simulink model "clutch"  (R2020a)
settings: Solver=VariableStepAuto  StartTime=0.0  StopTime=10.0  RelTol=1e-3
PostLoadFcn:
  | Fn=[0 0;1 0.8;2 1.6;3 1.6;4 1.6;5 1.6;6 0.8;7 0;8 0;9 0;10 0];
  | muk=1;
  | mus=1.5;
  | R=1;
  | Tin=[1 2;2 2;3 2;4 2;5 2;6 0;7 0;8 0;9 0;10 0];
  | Ie=1;
  | be=2;
  | Iv=5;
  | bv=1;
settings Model: Creator=Hp  LastModifiedBy=Hp

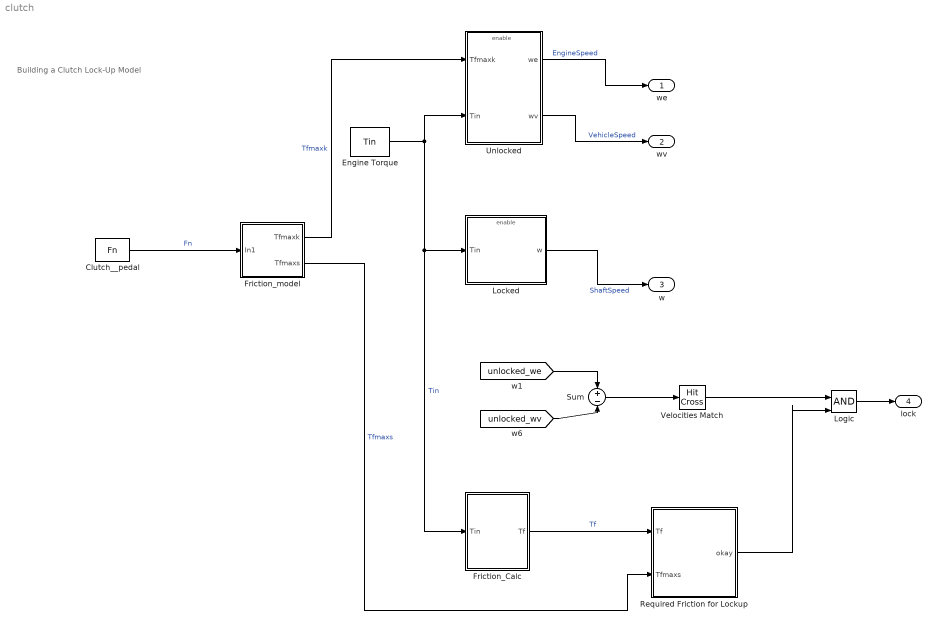
== system clutch ==
  note: Building a Clutch Lock-Up Model
  Clutch__pedal : FromWorkspace  VariableName=Fn
  Engine Torque : FromWorkspace  VariableName=Tin
  Friction_Calc : Subsystem
  Friction_model : Subsystem
  Locked : Subsystem
  Logic : Logic  IconShape=distinctive  OutDataTypeStr=boolean
  Required Friction for Lockup : Subsystem
  Sum : Sum  Inputs=+-  InputSameDT=on  SaturateOnIntegerOverflow=on  OutDataTypeStr=Inherit: Same as first input
  Unlocked : Subsystem
  Velocities Match : HitCross
  we : Outport  InitialOutput=0  VectorParamsAs1DForOutWhenUnconnected=off
  wv : Outport  Port=2  InitialOutput=0  VectorParamsAs1DForOutWhenUnconnected=off
  w : Outport  Port=3  InitialOutput=0  VectorParamsAs1DForOutWhenUnconnected=off
  lock : Outport  Port=4  InitialOutput=0  VectorParamsAs1DForOutWhenUnconnected=off
  wires:
  Clutch__pedal/1 -> Friction_model/1(In1)  "Fn"
  Engine Torque/1 -> Locked/1(Tin), Friction_Calc/1(Tin), Unlocked/2(Tin)  "Tin"
  Friction_model/1(Tfmaxk) -> Unlocked/1(Tfmaxk)  "Tfmaxk"
  Unlocked/1(we) -> we/1  "EngineSpeed"
  Unlocked/2(wv) -> wv/1  "VehicleSpeed"
  Locked/1(w) -> w/1  "ShaftSpeed"
  [unlocked_we] -> Sum/1
  Sum/1 -> Velocities Match/1
  Logic/1 -> lock/1
  [unlocked_wv] -> Sum/2
  Velocities Match/1 -> Logic/1
  Friction_model/2(Tfmaxs) -> Required Friction for Lockup/2(Tfmaxs)  "Tfmaxs"
  Friction_Calc/1(Tf) -> Required Friction for Lockup/1(Tf)  "Tf"
  Required Friction for Lockup/1(okay) -> Logic/2

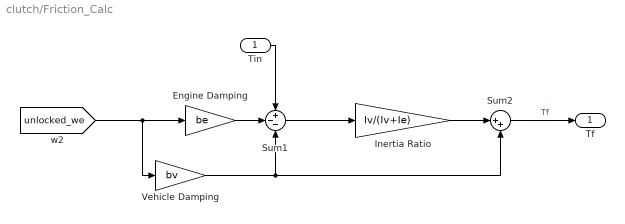
== system clutch/Friction_Calc ==
  Tin : Inport
  Engine Damping : Gain  Gain=be  SaturateOnIntegerOverflow=on  OutDataTypeStr=Inherit: Same as input  ParamDataTypeStr=Inherit: Same as input
  Inertia Ratio : Gain  Gain=Iv/(Iv+Ie)  SaturateOnIntegerOverflow=on  OutDataTypeStr=Inherit: Same as input  ParamDataTypeStr=Inherit: Same as input
  Sum1 : Sum  Inputs=+--  InputSameDT=on  SaturateOnIntegerOverflow=on  OutDataTypeStr=Inherit: Same as first input
  Sum2 : Sum  Inputs=|++  InputSameDT=on  SaturateOnIntegerOverflow=on  OutDataTypeStr=Inherit: Same as first input
  Vehicle Damping : Gain  Gain=bv  SaturateOnIntegerOverflow=on  OutDataTypeStr=Inherit: Same as input  ParamDataTypeStr=Inherit: Same as input
  Tf : Outport
  wires:
  Tin/1 -> Sum1/1
  [unlocked_we] -> Vehicle Damping/1, Engine Damping/1
  Inertia Ratio/1 -> Sum2/1
  Sum1/1 -> Inertia Ratio/1
  Sum2/1 -> Tf/1  "Tf"
  Engine Damping/1 -> Sum1/2
  Vehicle Damping/1 -> Sum2/2, Sum1/3

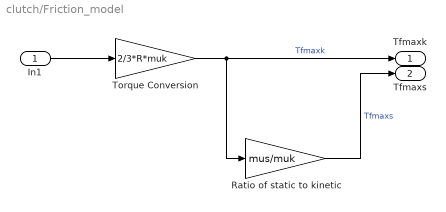
== system clutch/Friction_model ==
  In1 : Inport
  Ratio of static to kinetic : Gain  Gain=mus/muk  SaturateOnIntegerOverflow=on  OutDataTypeStr=Inherit: Same as input  ParamDataTypeStr=Inherit: Same as input
  Torque Conversion : Gain  Gain=2/3*R*muk  SaturateOnIntegerOverflow=on  OutDataTypeStr=Inherit: Same as input  ParamDataTypeStr=Inherit: Same as input
  Tfmaxk : Outport
  Tfmaxs : Outport  Port=2
  wires:
  In1/1 -> Torque Conversion/1
  Torque Conversion/1 -> Tfmaxk/1, Ratio of static to kinetic/1  "Tfmaxk"
  Ratio of static to kinetic/1 -> Tfmaxs/1  "Tfmaxs"

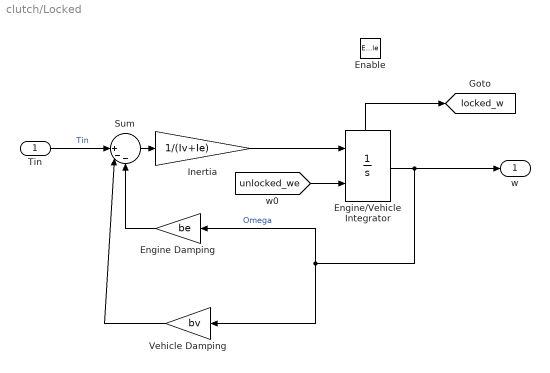
== system clutch/Locked ==
  Tin : Inport
  Enable : EnablePort
  Engine Damping : Gain  Gain=be  SaturateOnIntegerOverflow=on  OutDataTypeStr=Inherit: Same as input  ParamDataTypeStr=Inherit: Same as input
  Engine/Vehicle Integrator : Integrator  InitialConditionSource=external  ShowStatePort=on
  Inertia : Gain  Gain=1/(Iv+Ie)  SaturateOnIntegerOverflow=on  OutDataTypeStr=Inherit: Same as input  ParamDataTypeStr=Inherit: Same as input
  Sum : Sum  Inputs=||+--  InputSameDT=on  SaturateOnIntegerOverflow=on  OutDataTypeStr=Inherit: Same as first input
  Vehicle Damping : Gain  Gain=bv  SaturateOnIntegerOverflow=on  OutDataTypeStr=Inherit: Same as input  ParamDataTypeStr=Inherit: Same as input
  w : Outport  InitialOutput=0  VectorParamsAs1DForOutWhenUnconnected=off
  tag scope: locked_w=global
  wires:
  Inertia/1 -> Engine/Vehicle Integrator/1
  Engine/Vehicle Integrator/1 -> w/1, Engine Damping/1, Vehicle Damping/1  "Omega"
  Tin/1 -> Sum/1  "Tin"
  Vehicle Damping/1 -> Sum/2
  Engine Damping/1 -> Sum/3
  Engine/Vehicle Integrator/State -> [locked_w]
  Sum/1 -> Inertia/1
  [unlocked_we] -> Engine/Vehicle Integrator/2

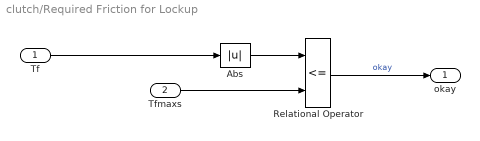
== system clutch/Required Friction for Lockup ==
  Tf : Inport
  Tfmaxs : Inport  Port=2
  Abs : Abs  SaturateOnIntegerOverflow=on
  Relational Operator : RelationalOperator  Operator=<=  OutDataTypeStr=boolean  RndMeth=Nearest  InputSameDT=on
  okay : Outport
  wires:
  Abs/1 -> Relational Operator/1
  Relational Operator/1 -> okay/1  "okay"
  Tfmaxs/1 -> Relational Operator/2
  Tf/1 -> Abs/1

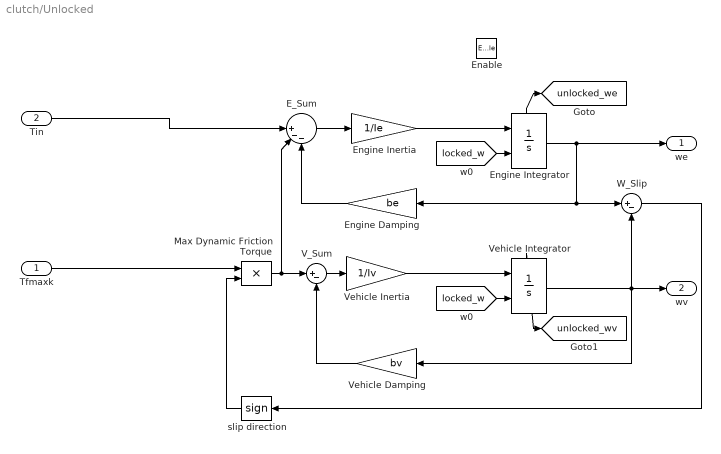
== system clutch/Unlocked ==
  Tfmaxk : Inport
  Tin : Inport  Port=2
  Enable : EnablePort
  E_Sum : Sum  Inputs=||+--  InputSameDT=on  SaturateOnIntegerOverflow=on  OutDataTypeStr=Inherit: Same as first input
  Engine Damping : Gain  Gain=be  SaturateOnIntegerOverflow=on  OutDataTypeStr=Inherit: Same as input  ParamDataTypeStr=Inherit: Same as input
  Engine Inertia : Gain  Gain=1/Ie  SaturateOnIntegerOverflow=on  OutDataTypeStr=Inherit: Same as input  ParamDataTypeStr=Inherit: Same as input
  Engine Integrator : Integrator  InitialConditionSource=external  ShowStatePort=on
  Max Dynamic Friction Torque : Product  InputSameDT=on  RndMeth=Zero  SaturateOnIntegerOverflow=on  OutDataTypeStr=Inherit: Same as first input
  V_Sum : Sum  Inputs=|+-  InputSameDT=on  SaturateOnIntegerOverflow=on  OutDataTypeStr=Inherit: Same as first input
  Vehicle Damping : Gain  Gain=bv  SaturateOnIntegerOverflow=on  OutDataTypeStr=Inherit: Same as input  ParamDataTypeStr=Inherit: Same as input
  Vehicle Inertia : Gain  Gain=1/Iv  SaturateOnIntegerOverflow=on  OutDataTypeStr=Inherit: Same as input  ParamDataTypeStr=Inherit: Same as input
  Vehicle Integrator : Integrator  InitialConditionSource=external  ShowStatePort=on
  W_Slip : Sum  Inputs=|+-  InputSameDT=on  SaturateOnIntegerOverflow=on  OutDataTypeStr=Inherit: Same as first input
  slip direction : Signum
  we : Outport  InitialOutput=0  VectorParamsAs1DForOutWhenUnconnected=off
  wv : Outport  Port=2  InitialOutput=0  VectorParamsAs1DForOutWhenUnconnected=off
  tag scope: unlocked_we=global, unlocked_wv=global
  wires:
  Engine Damping/1 -> E_Sum/3
  Vehicle Damping/1 -> V_Sum/2
  Vehicle Integrator/1 -> wv/1, W_Slip/2, Vehicle Damping/1
  Engine Integrator/1 -> we/1, Engine Damping/1, W_Slip/1
  Vehicle Inertia/1 -> Vehicle Integrator/1
  Max Dynamic Friction Torque/1 -> V_Sum/1, E_Sum/2
  Vehicle Integrator/State -> [unlocked_wv]
  slip direction/1 -> Max Dynamic Friction Torque/2
  Engine Inertia/1 -> Engine Integrator/1
  [locked_w] -> Engine Integrator/2
  [locked_w] -> Vehicle Integrator/2
  W_Slip/1 -> slip direction/1
  V_Sum/1 -> Vehicle Inertia/1
  Engine Integrator/State -> [unlocked_we]
  E_Sum/1 -> Engine Inertia/1
  Tin/1 -> E_Sum/1
  Tfmaxk/1 -> Max Dynamic Friction Torque/1
